simulink model "testIf"  (R2022a)
settings: Solver=VariableStepAuto  StartTime=0.0  StopTime=200  RelTol=1e-3
libraries: simulink x1
settings Model: Creator=janbantle  LastModifiedBy=janbantle

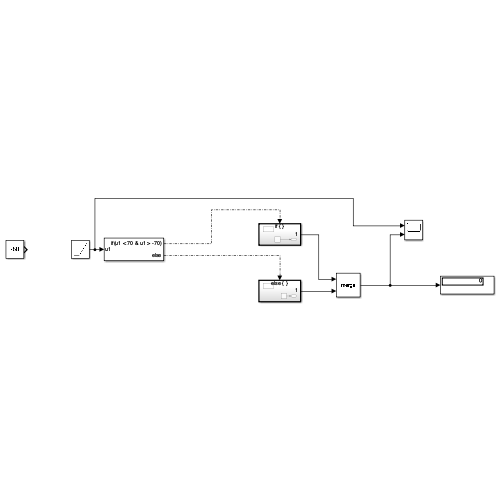
[thumbnail: Simulink's stored preview of the top-level diagram]
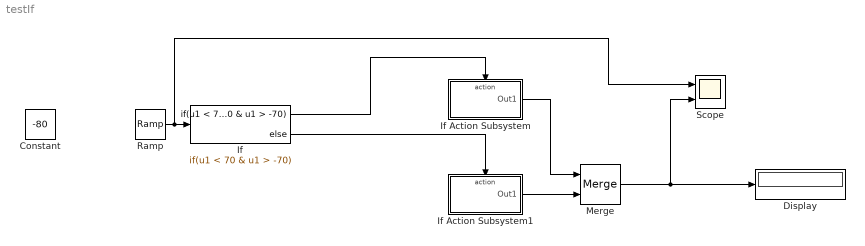
== system testIf ==
  Constant : Constant  Value=-80
  Display : Display
  If : If  IfExpression=u1 < 70 & u1 > -70
  If Action Subsystem : Subsystem  TreatAsAtomicUnit=on
  If Action Subsystem1 : Subsystem  TreatAsAtomicUnit=on
  Merge : Merge
  Ramp : simulink/Sources/Ramp  slope=1  start=0  InitialOutput=-100
  Scope : Scope  NumInputPorts=2
  wires:
  If/1 -> If Action Subsystem/Action
  If/2 -> If Action Subsystem1/Action
  If Action Subsystem/1(Out1) -> Merge/1
  If Action Subsystem1/1(Out1) -> Merge/2
  Merge/1 -> Scope/2, Display/1
  Ramp/1 -> Scope/1, If/1

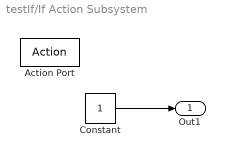
== system testIf/If Action Subsystem ==
  Action Port : ActionPort  ActionPortLabel=if(u1 < 70 & u1 > -70)
  Constant : Constant
  Out1 : Outport
  wires:
  Constant/1 -> Out1/1

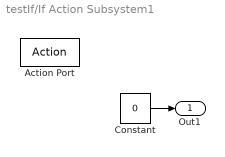
== system testIf/If Action Subsystem1 ==
  Action Port : ActionPort  ActionPortLabel=else
  Constant : Constant  Value=0
  Out1 : Outport
  wires:
  Constant/1 -> Out1/1
